simulink model "dealgaefier"  (R2024a)
settings: Solver=VariableStepAuto  StartTime=0.0  StopTime=10.0  RelTol=1e-3
settings Model: Creator=micah  LastModifiedBy=micah

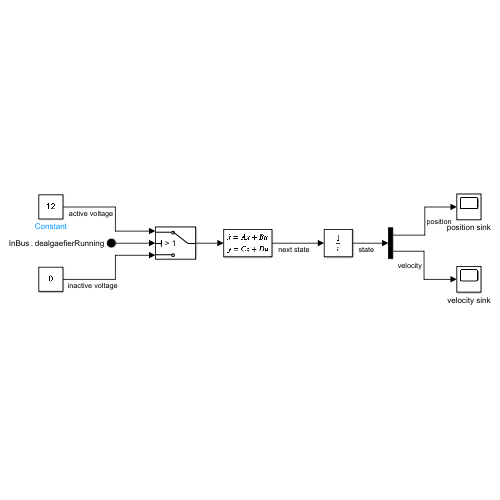
[thumbnail: Simulink's stored preview of the top-level diagram]
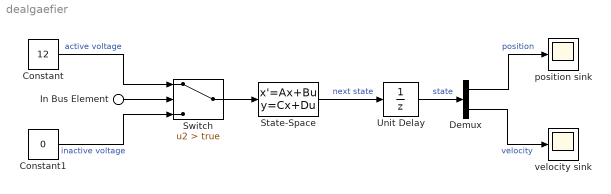
== system dealgaefier ==
  In Bus Element : Inport  PortName=InBus  Element=dealgaefierRunning
  Constant : Constant  Value=12  OutDataTypeStr=double
  Constant1 : Constant  Value=0  OutDataTypeStr=double
  Demux : Demux  Outputs=2
  State-Space : StateSpace  InitialCondition=0
  Switch : Switch  Criteria=u2 > Threshold  Threshold=true  SaturateOnIntegerOverflow=off  InputSameDT=off
  Unit Delay : UnitDelay  SampleTime=-1  HasFrameUpgradeWarning=on
  position sink : Scope
  velocity sink : Scope
  wires:
  In Bus Element/1 -> Switch/2
  Constant/1 -> Switch/1  "active voltage"
  Constant1/1 -> Switch/3  "inactive voltage"
  Switch/1 -> State-Space/1
  State-Space/1 -> Unit Delay/1  "next state"
  Unit Delay/1 -> Demux/1  "state"
  Demux/2 -> velocity sink/1  "velocity"
  Demux/1 -> position sink/1  "position"
